simulink model "Vehicle_model"  (R2018a)
settings: Solver=FixedStepAuto  StartTime=0.0  StopTime=40  FixedStep=1e-3  RelTol=1e-2
model workspace (MAT data in the model file):
  Af = 4
  Cd = 0.3
  DrCycles.C505 = [0 1 2 3 4 5 6 7 8 9 10 11 ... (1012 elements, 506x2)]
  DrCycles.FTP = [0 1 2 3 4 5 6 7 8 9 10 11 ... (4956 elements, 2478x2)]
  DrCycles.UDDS = [0 1 2 3 4 5 6 7 8 9 10 11 ... (2746 elements, 1373x2)]
  DrCycles.HWFET = [0 1 2 3 4 5 6 7 8 9 10 11 ... (1532 elements, 766x2)]
  DrCycles.US06 = [0 1 2 3 4 5 6 7 8 9 10 11 ... (1194 elements, 597x2)]
  DrCycles.US06City = [0 1 2 3 4 5 6 7 8 9 10 11 ... (466 elements, 233x2)]
  DrCycles.US06Hwy = [0 1 2 3 4 5 6 7 8 9 10 11 ... (742 elements, 371x2)]
  I = 1
  Kbr = 5000
  P = 20
  Sig = Simulink.Signal
  Sig.DataType = 'auto'
  Sig.Dimensions = -1
  Sig.DimensionsMode = 'auto'
  Sig.Complexity = 'auto'
  Sig.SampleTime = -1
  Sig.SamplingMode = 'auto'
  TimeHWFET = 765
  TimeUDDS = 1372
  TimeUS06 = 596
  axle_b = 10
  axle_k = 5000
  bevAxle_wc = 400
  bevNp = 2
  bevNs = 30
  diffRatio = 3.4
  diffRatio1 = 3.4
  motorMaxTorqueNm = [500 500 500 500 500 500 416.666666667 357.142857143 312.5 277.777777778 250 227.272727273 208.333333333 192.307692308 178.571428571 166.666666667]
  motorMaxTorqueNm2 = [220 220 220 220 220 220 198 176 165 154 143 132 121 110 88 66]
  motorSpeedRadPs = [0 40 80 120 160 200 240 280 320 360 400 440 480 520 560 600]
  motorSpeedRadPs2 = [0 84 168 251 335 419 503 586 670 754 838 922 1005 1089 1173 1361]
  vehicleMass = 1500
  wheelRadius = 0.35
undefined symbols (not defined in the file or in its folder): sigbuilder_block, W_h_o, W_i_h
libraries: simulink x4, autolibdatasheetbattery x2, autolibmappedmotor x2, autolibsharedcoupling x2, autolibshareddiff x2, autolibshared x2, Wheels_Driver_VehDyn_Lib x2
settings Model: PauseTimes=2  Creator=ogden.michael  LastModifiedBy=yassi
settings SolverCC: ZeroCrossAlgorithm=Adaptive
settings DebuggingCC: AlgebraicLoopMsg=none  IgnoredZcDiagnostic=none
settings CodeAppCC: StateflowObjectComments=on
settings SimscapeCC: SimscapeNormalizeSystem=off

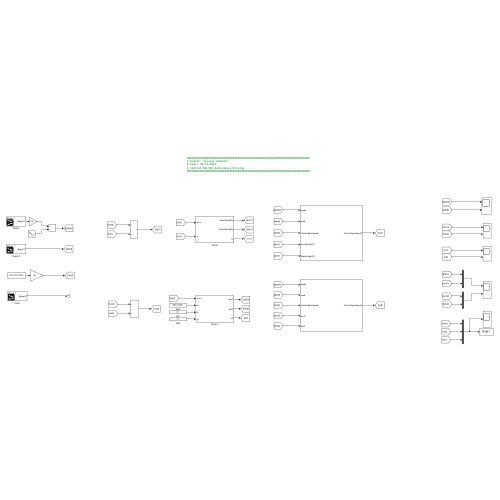
[thumbnail: Simulink's stored preview of the top-level diagram]
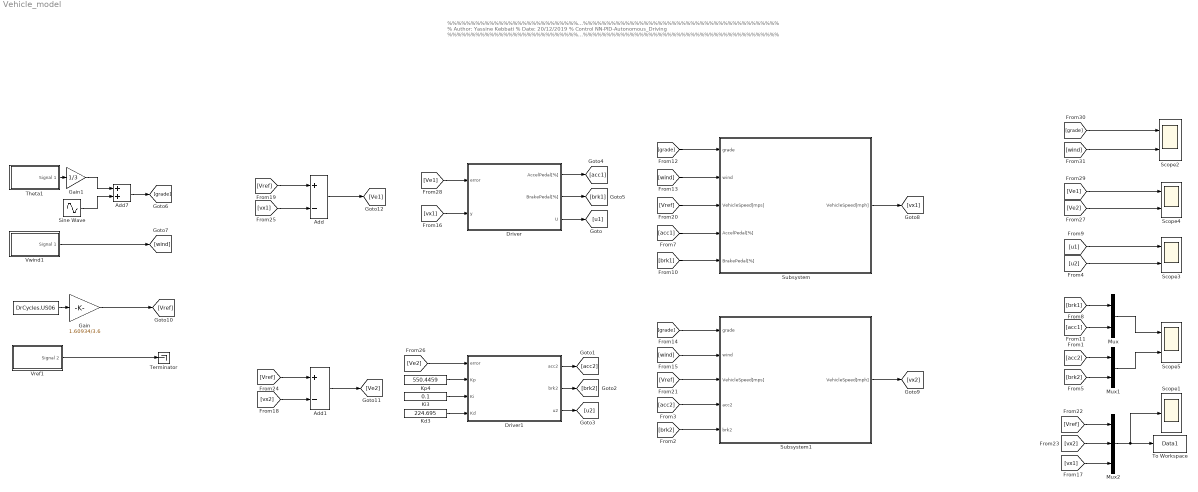
== system Vehicle_model ==
  note: %%%%%%%%%%%%%%%%%%%%%%%%%%%%%%%%%%%%%%%%%%%%%%%%%%%%%%%%%%%%%%%%%%%%%%%%%%%
      | % Author: Yassine Kebbati
      | % Date: 20/12/2019
      | % Control NN-PID-Autonomous_Driving
      | %%%%%%%%%%%%%%%%%%%%%%%%%%%%%%%%%%%%%%%%%%%%%%%%%%%%%%%%%%%%%%%%%%%%%%%%%%%
  " " : FromWorkspace  Tag=DriveCycle  VariableName=DrCycles.US06
  Add : Sum  Inputs=+-
  Add1 : Sum  Inputs=+-
  Add7 : Sum
  Driver : Subsystem  AncestorBlock=Wheels_Driver_VehDyn_Lib/Driver
  Driver1 : Subsystem  AncestorBlock=Wheels_Driver_VehDyn_Lib/Driver
  Gain : Gain  Gain=1.60934/3.6
  Gain1 : Gain  Gain=1/3
  Kd3 : Constant  Value=224.695
  Ki3 : Constant  Value=0.1
  Kp4 : Constant  Value=550.4459
  Mux : Mux  Inputs=2
  Mux1 : Mux  Inputs=2
  Mux2 : Mux  Inputs=3
  Scope1 : Scope
  Scope{2..5} (4 alike) : Scope  NumInputPorts=2
  Sine Wave : Sin  Amplitude=4  Frequency=0.2  SampleTime=0
  Subsystem : Subsystem
  Subsystem1 : Subsystem
  Terminator : Terminator
  Theta1 : Subsystem  Tag=STV Subsys  LoadFcn=sigbuilder_block('load');  StartFcn=sigbuilder_block('start');  StopFcn=sigbuilder_block('stop');  ClipboardFcn=sigbuilder_block('clipboard');  mask(Sigbuilder block){tuvar=[0:10]}
      mask help: Simulink:masks:SigbuilderBlock_MD
      mask init:
      | if ~strcmp(get_param(bdroot(gcbh),'SimulationStatus'),'stopped') tuvar = sigbuilder_block('maskInit'); end
      settings: CopyFcn=sigbuilder_block('copy');  DeleteFcn=sigbuilder_block('delete');  ModelCloseFcn=sigbuilder_block('modelClose');  PreSaveFcn=sigbuilder_block('preSave');  PauseFcn=sigbuilder_block('pause');  ContinueFcn=sigbuilder_block('continue');  NameChangeFcn=sigbuilder_block('namechange');  OpenFcn=sigbuilder_block('open',[6 30 1428 681.75 ]);  CloseFcn=sigbuilder_block('close');
      mask Display: plot(0, 0, 100, 100,[2, 2, 32, 32, 2], [68, 8, 8, 68, 68],[32, 2], [38, 38], [32, 19, 2],[53, 60, 44], [32, 17, 17, 2],[16, 16, 31, 31]);txt = getActiveGroup(gcbh);text(2, 100, txt,'verticalAlignment', 'top');
  To Workspace : ToWorkspace  VariableName=Data1  SaveFormat=Timeseries  SampleTime=-1
  Vref1 : Subsystem  Tag=STV Subsys  LoadFcn=sigbuilder_block('load');  StartFcn=sigbuilder_block('start');  StopFcn=sigbuilder_block('stop');  ClipboardFcn=sigbuilder_block('clipboard');  mask(Sigbuilder block){tuvar=[0:10]}
      mask help: Simulink:masks:SigbuilderBlock_MD
      mask init:
      | if ~strcmp(get_param(bdroot(gcbh),'SimulationStatus'),'stopped') tuvar = sigbuilder_block('maskInit'); end
      settings: CopyFcn=sigbuilder_block('copy');  DeleteFcn=sigbuilder_block('delete');  ModelCloseFcn=sigbuilder_block('modelClose');  PreSaveFcn=sigbuilder_block('preSave');  PauseFcn=sigbuilder_block('pause');  ContinueFcn=sigbuilder_block('continue');  NameChangeFcn=sigbuilder_block('namechange');  OpenFcn=sigbuilder_block('open',[6 51.75 1428 641.25 ]);  CloseFcn=sigbuilder_block('close');
      mask Display: plot(0, 0, 100, 100,[2, 2, 32, 32, 2], [68, 8, 8, 68, 68],[32, 2], [38, 38], [32, 19, 2],[53, 60, 44], [32, 17, 17, 2],[16, 16, 31, 31]);txt = getActiveGroup(gcbh);text(2, 100, txt,'verticalAlignment', 'top');
  Vwind1 : Subsystem  Tag=STV Subsys  LoadFcn=sigbuilder_block('load');  StartFcn=sigbuilder_block('start');  StopFcn=sigbuilder_block('stop');  ClipboardFcn=sigbuilder_block('clipboard');  mask(Sigbuilder block){tuvar=[0:10]}
      mask help: Simulink:masks:SigbuilderBlock_MD
      mask init:
      | if ~strcmp(get_param(bdroot(gcbh),'SimulationStatus'),'stopped') tuvar = sigbuilder_block('maskInit'); end
      settings: CopyFcn=sigbuilder_block('copy');  DeleteFcn=sigbuilder_block('delete');  ModelCloseFcn=sigbuilder_block('modelClose');  PreSaveFcn=sigbuilder_block('preSave');  PauseFcn=sigbuilder_block('pause');  ContinueFcn=sigbuilder_block('continue');  NameChangeFcn=sigbuilder_block('namechange');  OpenFcn=sigbuilder_block('open',[6 30 1428 681.75 ]);  CloseFcn=sigbuilder_block('close');
      mask Display: plot(0, 0, 100, 100,[2, 2, 32, 32, 2], [68, 8, 8, 68, 68],[32, 2], [38, 38], [32, 19, 2],[53, 60, 44], [32, 17, 17, 2],[16, 16, 31, 31]);txt = getActiveGroup(gcbh);text(2, 100, txt,'verticalAlignment', 'top');
  wires:
  [grade] -> Subsystem/1(grade)
  Sine Wave/1 -> Add7/2
  Theta1/1(Signal 1) -> Gain1/1
  [Ve1] -> Driver/1(" error")
  Gain1/1 -> Add7/1
  [wind] -> Subsystem/2(wind)
  Kp4/1 -> Driver1/2(Kp)
  Ki3/1 -> Driver1/3(Ki)
  Kd3/1 -> Driver1/4(Kd)
  Mux/1 -> Scope5/1
  Mux1/1 -> Scope5/2
  [Ve2] -> Scope4/2
  Mux2/1 -> To Workspace/1, Scope1/1
  [vx2] -> Add1/2
  [vx1] -> Driver/2(" y")
  [Vref] -> Add/1
  Vwind1/1(Signal 1) -> [wind]
  Add7/1 -> [grade]
  Driver1/1(acc2) -> [acc2]
  Driver1/2(brk2) -> [brk2]
  [acc2] -> Subsystem1/4(acc2)
  [acc2] -> Mux1/1
  [brk2] -> Subsystem1/5(brk2)
  [brk2] -> Mux1/2
  [u2] -> Scope3/2
  Driver1/3(u2) -> [u2]
  Driver/3(U) -> [u1]
  [u1] -> Scope3/1
  Driver/2(BrakePedal[%]) -> [brk1]
  [brk1] -> Mux/1
  [brk1] -> Subsystem/5(BrakePedal[%])
  Driver/1(AccelPedal[%]) -> [acc1]
  [acc1] -> Subsystem/4(AccelPedal[%])
  [acc1] -> Mux/2
  [grade] -> Subsystem1/1(grade)
  [wind] -> Subsystem1/2(wind)
  Subsystem/1(VehicleSpeed[mph]) -> [vx1]
  [vx1] -> Mux2/3
  Subsystem1/1(VehicleSpeed[mph]) -> [vx2]
  [Vref] -> Subsystem/3(VehicleSpeed[mps])
  [Vref] -> Subsystem1/3(VehicleSpeed[mps])
  [Vref] -> Mux2/1
  [vx2] -> Mux2/2
  [Vref] -> Add1/1
  [vx1] -> Add/2
  Add1/1 -> [Ve2]
  [Ve2] -> Driver1/1(" error")
  Add/1 -> [Ve1]
  [Ve1] -> Scope4/1
  [grade] -> Scope2/1
  [wind] -> Scope2/2
  " "/1 -> Gain/1
  Vref1/1(Signal 2) -> Terminator/1
  Gain/1 -> [Vref]

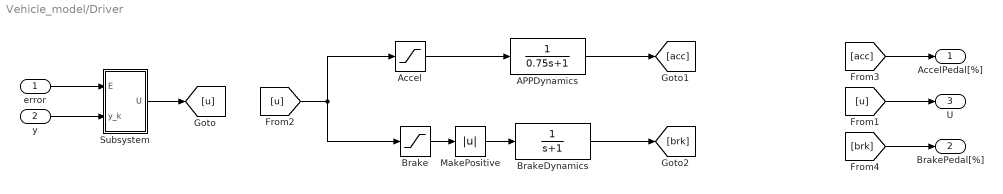
== system Vehicle_model/Driver ==
  " error" : Inport
  " y" : Inport  Port=2
  APPDynamics : TransferFcn  Denominator=[0.75 1]
  Accel : Saturate  UpperLimit=100  LowerLimit=0
  Brake : Saturate  UpperLimit=0  LowerLimit=-100
  BrakeDynamics : TransferFcn  Denominator=[1 1]
  MakePositive : Abs
  Subsystem : Subsystem
  AccelPedal[%] : Outport  VectorParamsAs1DForOutWhenUnconnected=off
  BrakePedal[%] : Outport  Port=2  VectorParamsAs1DForOutWhenUnconnected=off
  U : Outport  Port=3  VectorParamsAs1DForOutWhenUnconnected=off
  wires:
  MakePositive/1 -> BrakeDynamics/1
  " error"/1 -> Subsystem/1(E)
  Accel/1 -> APPDynamics/1
  Brake/1 -> MakePositive/1
  " y"/1 -> Subsystem/2(y_k)
  BrakeDynamics/1 -> [brk]
  APPDynamics/1 -> [acc]
  [u] -> Accel/1, Brake/1
  Subsystem/1(U) -> [u]
  [u] -> U/1
  [acc] -> AccelPedal[%]/1
  [brk] -> BrakePedal[%]/1

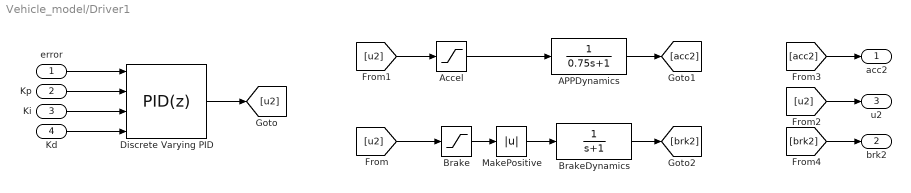
== system Vehicle_model/Driver1 ==
  " error" : Inport
  Kp : Inport  Port=2
  Ki : Inport  Port=3
  Kd : Inport  Port=4
  APPDynamics : TransferFcn  Denominator=[0.75 1]
  Accel : Saturate  UpperLimit=100  LowerLimit=0
  Brake : Saturate  UpperLimit=0  LowerLimit=-100
  BrakeDynamics : TransferFcn  Denominator=[1 1]
  Discrete Varying PID : simulink/Continuous/PID Controller  Controller=PID  Form=Parallel  TimeDomain=Discrete-time  SampleTime=-1  IntegratorMethod=Forward Euler  ControllerParametersSource=external  P=1  I=1  D=0  N=100  UseFilter=off  TunerSelectOption=Transfer Function Based (PID Tuner App)  InitialConditionSource=internal  InitialConditionForIntegrator=0  InitialConditionForFilter=0  DifferentiatorICPrevScaledInput=0  ExternalReset=none  TrackingMode=off  Kt=1  LimitOutput=off  UpperSaturationLimit=100  LowerSaturationLimit=-100  LinearizeAsGain=on  AntiWindupMode=none  Kb=1  POutMin=[]  POutMax=[]  IOutMin=[]  IOutMax=[]  DOutMin=[]  DOutMax=[]  NOutMin=[]  NOutMax=[]  SumOutMin=[]  SumOutMax=[]  SaturationOutMin=[]  SaturationOutMax=[]  PParamMin=[]  PParamMax=[]  IParamMin=[]  IParamMax=[]  DParamMin=[]  DParamMax=[]  NParamMin=[]  NParamMax=[]  KbParamMin=[]  KbParamMax=[]  KtParamMin=[]  KtParamMax=[]  KbOutMin=[]  KbOutMax=[]  KtOutMin=[]  KtOutMax=[]  IntegratorOutMin=[]  IntegratorOutMax=[]  FilterOutMin=[]  FilterOutMax=[]  SumI1OutMin=[]  SumI1OutMax=[]  SumI2OutMin=[]  SumI2OutMax=[]  SumI3OutMin=[]  SumI3OutMax=[]  SumDOutMin=[]  SumDOutMax=[]  DifferentiatorOutMin=[]  DifferentiatorOutMax=[]  FilterDiffOutCoefMin=[]  FilterDiffOutCoefMax=[]  ReciprocalOutMin=[]  ReciprocalOutMax=[]  SumDenOutMin=[]  SumDenOutMax=[]  SumNumOutMin=[]  SumNumOutMax=[]  DivideOutMin=[]  DivideOutMax=[]  IntegratorContinuousStateAttributes=''  IntegratorStateMustResolveToSignalObject=off  IntegratorRTWStateStorageClass=Auto  FilterContinuousStateAttributes=''  FilterStateMustResolveToSignalObject=off  FilterRTWStateStorageClass=Auto
  MakePositive : Abs
  acc2 : Outport  VectorParamsAs1DForOutWhenUnconnected=off
  brk2 : Outport  Port=2  VectorParamsAs1DForOutWhenUnconnected=off
  u2 : Outport  Port=3  VectorParamsAs1DForOutWhenUnconnected=off
  wires:
  MakePositive/1 -> BrakeDynamics/1
  " error"/1 -> Discrete Varying PID/1
  Accel/1 -> APPDynamics/1
  Kp/1 -> Discrete Varying PID/2
  Kd/1 -> Discrete Varying PID/4
  Ki/1 -> Discrete Varying PID/3
  Brake/1 -> MakePositive/1
  BrakeDynamics/1 -> [brk2]
  APPDynamics/1 -> [acc2]
  Discrete Varying PID/1 -> [u2]
  [u2] -> Brake/1
  [u2] -> Accel/1
  [u2] -> u2/1
  [acc2] -> acc2/1
  [brk2] -> brk2/1

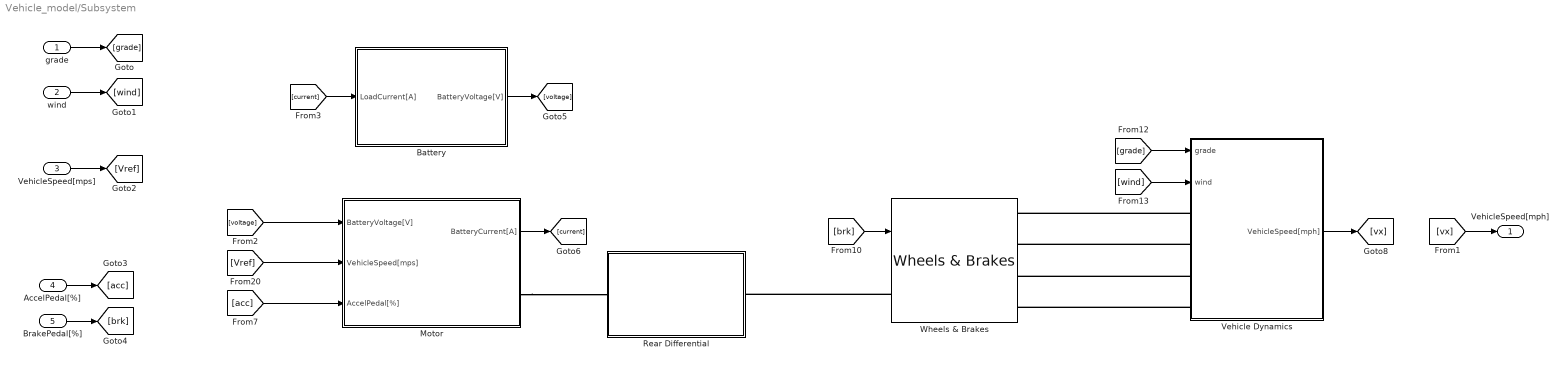
== system Vehicle_model/Subsystem ==
  grade : Inport
  wind : Inport  Port=2
  VehicleSpeed[mps] : Inport  Port=3
  AccelPedal[%] : Inport  Port=4
  BrakePedal[%] : Inport  Port=5
  Battery : Subsystem
  Motor : Subsystem
  Rear Differential : Subsystem
  Vehicle Dynamics : Subsystem  AncestorBlock=Wheels_Driver_VehDyn_Lib/Vehicle Dynamics
  "Wheels & Brakes " : Wheels_Driver_VehDyn_Lib/Wheels & Brakes  SystemSampleTime=-1  Latency=0  AutoFrameSizeCalculation=off
      link override BrakeGain: Gain=Kbr
      link override Longitudinal Wheel - Disk Brake: Re=0.32995  Lrel=0.32995  rollingType=Magic Formula  Iyy=0.798  UNLOADED_RADIUS=0.32995  num_pads=2
      link override Longitudinal Wheel - Disk Brake1: Iyy=0.798  Lrel=0.32995  Re=0.32995  rollingType=Magic Formula  UNLOADED_RADIUS=0.32995
  VehicleSpeed[mph] : Outport
  wires:
  [wind] -> Vehicle Dynamics/2(wind)
  [current] -> Battery/1(LoadCurrent[A])
  [voltage] -> Motor/1(BatteryVoltage[V])
  [grade] -> Vehicle Dynamics/1(grade)
  [vx] -> VehicleSpeed[mph]/1
  [brk] -> "Wheels & Brakes "/1
  [Vref] -> Motor/2(VehicleSpeed[mps])
  [acc] -> Motor/3(AccelPedal[%])
  Vehicle Dynamics/1(VehicleSpeed[mph]) -> [vx]
  grade/1 -> [grade]
  wind/1 -> [wind]
  VehicleSpeed[mps]/1 -> [Vref]
  AccelPedal[%]/1 -> [acc]
  BrakePedal[%]/1 -> [brk]
  Battery/1(BatteryVoltage[V]) -> [voltage]
  Motor/1(BatteryCurrent[A]) -> [current]
  connections:
  Motor/RConn1 -- Rear Differential/LConn1
  Vehicle Dynamics/LConn4 -- "Wheels & Brakes "/RConn4
  Vehicle Dynamics/LConn2 -- "Wheels & Brakes "/RConn2
  Vehicle Dynamics/LConn1 -- "Wheels & Brakes "/RConn1
  Vehicle Dynamics/LConn3 -- "Wheels & Brakes "/RConn3
  "Wheels & Brakes "/LConn1 -- Rear Differential/RConn1

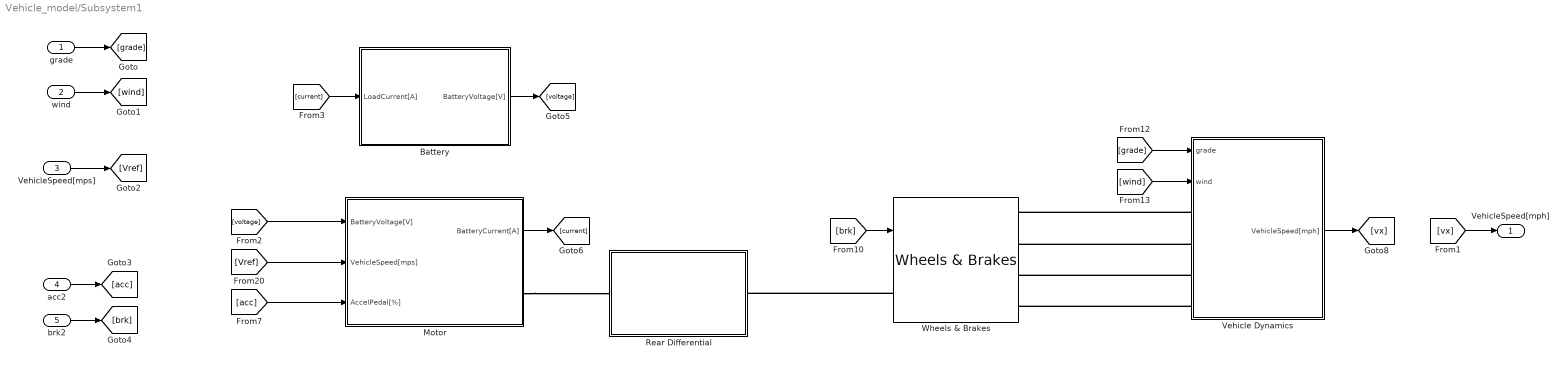
== system Vehicle_model/Subsystem1 ==
  grade : Inport
  wind : Inport  Port=2
  VehicleSpeed[mps] : Inport  Port=3
  acc2 : Inport  Port=4
  brk2 : Inport  Port=5
  Battery : Subsystem
  Motor : Subsystem
  Rear Differential : Subsystem
  Vehicle Dynamics : Subsystem  AncestorBlock=Wheels_Driver_VehDyn_Lib/Vehicle Dynamics
  "Wheels & Brakes " : Wheels_Driver_VehDyn_Lib/Wheels & Brakes  SystemSampleTime=-1  Latency=0  AutoFrameSizeCalculation=off
      link override BrakeGain: Gain=Kbr
      link override Longitudinal Wheel - Disk Brake: Re=0.32995  Lrel=0.32995  rollingType=Magic Formula  Iyy=0.798  UNLOADED_RADIUS=0.32995  num_pads=2
      link override Longitudinal Wheel - Disk Brake1: Iyy=0.798  Lrel=0.32995  Re=0.32995  rollingType=Magic Formula  UNLOADED_RADIUS=0.32995
  VehicleSpeed[mph] : Outport
  wires:
  [vx] -> VehicleSpeed[mph]/1
  wind/1 -> [wind]
  [Vref] -> Motor/2(VehicleSpeed[mps])
  [grade] -> Vehicle Dynamics/1(grade)
  [acc] -> Motor/3(AccelPedal[%])
  [current] -> Battery/1(LoadCurrent[A])
  VehicleSpeed[mps]/1 -> [Vref]
  brk2/1 -> [brk]
  Motor/1(BatteryCurrent[A]) -> [current]
  [voltage] -> Motor/1(BatteryVoltage[V])
  Vehicle Dynamics/1(VehicleSpeed[mph]) -> [vx]
  [brk] -> "Wheels & Brakes "/1
  [wind] -> Vehicle Dynamics/2(wind)
  grade/1 -> [grade]
  acc2/1 -> [acc]
  Battery/1(BatteryVoltage[V]) -> [voltage]
  connections:
  Motor/RConn1 -- Rear Differential/LConn1
  Vehicle Dynamics/LConn4 -- "Wheels & Brakes "/RConn4
  Vehicle Dynamics/LConn3 -- "Wheels & Brakes "/RConn3
  "Wheels & Brakes "/LConn1 -- Rear Differential/RConn1
  Vehicle Dynamics/LConn1 -- "Wheels & Brakes "/RConn1
  Vehicle Dynamics/LConn2 -- "Wheels & Brakes "/RConn2

== system Vehicle_model/Theta1 ==
  Demux : Demux  Tag=STV Demux  Outputs=1
      settings: DisplayOption=none
  FromWs : FromWorkspace  Tag=STV FromWs  VariableName=tuvar
      SigBuilderData=|
      | common.afterFinalStr = 'Extrapolate'
      | common.sampleTime = 0
      | dataSet.timeRange = [0 100]
      | dataSet.name = 'Group 1'
      | sbobj.Groups.Name = 'Group 1'
      | sbobj.Groups.Signals.Name = 'Signal 1'
      | sbobj.Groups.Signals.XData = [0 1 2 3 4 5 6 7 8 9 10 11 12 13 14 15 16 17 18 19 20 21 22 23 24 25 26 27 28 29 30 31 32 33 34 35 36 37 38 39 40 41 42 43 44 45 46 47 48 49 50 51 52 53 54 55 56 57 58 59 60 61 62 63 64 65 66 67 68 69 70 71 72 73 74 75 76 77 78 79 80 81 82 83 84 85 86 87 88 89 90 91 92 93 94 95 96 97 98 100]
      | sbobj.Groups.Signals.YData = [0 0 0 0 0 0 0 0.05 0.15 0.2 0.5 1 2 3 4 5 6 7 8 9 10 11 12 13 14 14.5 14.8 15 15 15 15 15 15 15 14.95 14.7 14.45 14.1 13.15 11.85 11 9.95 8.7 8.15 7.35 6 4.6 3.55 2.25 1.35 0.75 0.15 0 0 0 0 0 0 0 0 -0.15 -0.4 -1.15 -2 -3 -4 -5 -6 -6.65 -7.45 -7.9 -8 -8 -8 -8 -8 -8 -8 -8 -8 -7.8 -7.55 -7.45 -7.15 -6.85 -6.5 -6 -5.5 -5.25 -5.2 -5.2 -5.15 -5 -5 -5 -5 -5 -5 -5 -5]
      | sbobj.Groups.TimeRange = [0 100]
  Signal 1 : Outport  Tag=STV Outport
  wires:
  Demux/1 -> Signal 1/1
  FromWs/1 -> Demux/1

== system Vehicle_model/Vref1 ==
  Demux : Demux  Tag=STV Demux  Outputs=1
      settings: DisplayOption=none
  FromWs : FromWorkspace  Tag=STV FromWs  VariableName=tuvar
      SigBuilderData=|
      | common.afterFinalStr = 'Extrapolate'
      | common.sampleTime = 0
      | dataSet.timeRange = [0 99]
      | dataSet.name = 'Group 1'
      | sbobj.Groups.Name = 'Group 1'
      | sbobj.Groups.Signals.Name = 'Signal 2'
      | sbobj.Groups.Signals.XData = [0 1 2 3 4 5 6 7 8 9 10 11 12 13 14 15 16 17 18 19 20 21 22 23 24 25 26 27 28 29 30 31 32 33 34 35 36 37 38 39 40 41 42 43 44 45 46 47 48 49 50 51 52 53 54 55 56 57 58 59 60 61 62 63 64 65 66 67 68 69 70 71 72 73 74 75 76 77 78 79 80 81 82 83 84 85 86 87 88 89 90 91 92 93 94 95 96 97 98 99]
      | sbobj.Groups.Signals.YData = [5 5 5 5 5 5 5 5 5 5 5 5 5 5 5 5 5 5 5 5 15 15 15 15 15 15 15 15 15 15 15 15 15 15 15 15 15 15 15 15 30 30 30 30 30 30 30 30 30 30 30 30 30 30 30 30 30 30 30 30 20 20 20 20 20 20 20 20 20 20 20 20 20 20 20 20 20 20 20 20 10 10 10 10 10 10 10 10 10 10 10 10 10 10 10 10 10 10 10 10]
      | sbobj.Groups.TimeRange = [0 99]
  Signal 2 : Outport  Tag=STV Outport
  wires:
  FromWs/1 -> Demux/1
  Demux/1 -> Signal 2/1

== system Vehicle_model/Vwind1 ==
  Demux : Demux  Tag=STV Demux  Outputs=1
      settings: DisplayOption=none
  FromWs : FromWorkspace  Tag=STV FromWs  VariableName=tuvar
      SigBuilderData=|
      | common.afterFinalStr = 'Extrapolate'
      | common.sampleTime = 0
      | dataSet.timeRange = [0 100]
      | dataSet.name = 'Group 1'
      | sbobj.Groups.Name = 'Group 1'
      | sbobj.Groups.Signals.Name = 'Signal 1'
      | sbobj.Groups.Signals.XData = [0 1 2 3 4 5 6 7 8 9 10 11 12 13 14 15 16 17 18 19 20 21 22 23 24 25 26 27 28 29 30 31 32 33 34 35 36 37 38 39 40 41 42 43 44 45 46 47 48 49 50 51 52 53 54 55 56 57 58 59 60 61 62 63 64 65 66 67 68 69 70 71 72 73 74 75 76 77 78 79 80 81 82 83 84 85 86 87 88 89 90 91 92 93 94 95 96 97 98 100]
      | sbobj.Groups.Signals.YData = [-8 -8 -8 -8 -8 -8 -8 -8 -8 -8 -8 -8 -8 -8 -8 -8 -8 -8 -8 -8 -2 -2 -2 -2 -2 -2 -2 -2 -2 -2 -2 -2 -2 -2 -2 -2 -2 -2 -2 -2 10 10 10 10 10 10 10 10 10 10 10 10 10 10 10 10 10 10 10 10 15 15 15 15 15 15 15 15 15 15 15 15 15 15 15 15 15 15 15 15 5 5 5 5 5 5 5 5 5 5 5 5 5 5 5 5 5 5 5 5]
      | sbobj.Groups.TimeRange = [0 100]
  Signal 1 : Outport  Tag=STV Outport
  wires:
  FromWs/1 -> Demux/1
  Demux/1 -> Signal 1/1

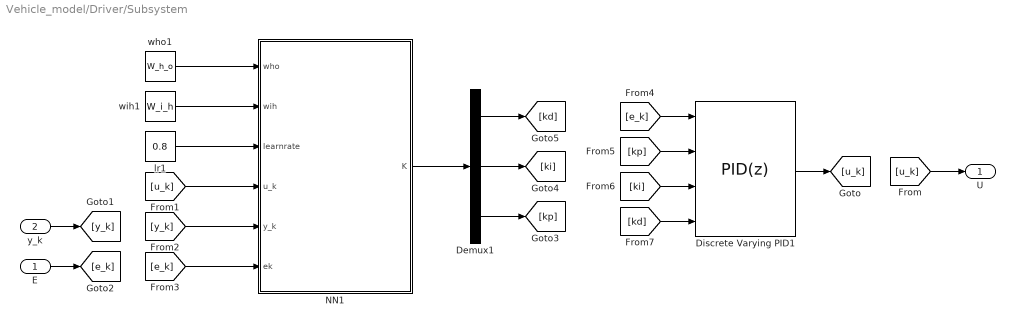
== system Vehicle_model/Driver/Subsystem ==
  E : Inport
  y_k : Inport  Port=2
  Demux1 : Demux  Outputs=3
  Discrete Varying PID1 : simulink/Continuous/PID Controller  Controller=PID  Form=Parallel  TimeDomain=Discrete-time  SampleTime=-1  IntegratorMethod=Forward Euler  ControllerParametersSource=external  P=1  I=1  D=0  N=100  UseFilter=off  TunerSelectOption=Transfer Function Based (PID Tuner App)  InitialConditionSource=internal  InitialConditionForIntegrator=0  InitialConditionForFilter=0  DifferentiatorICPrevScaledInput=0  ExternalReset=none  TrackingMode=off  Kt=1  LimitOutput=off  UpperSaturationLimit=100  LowerSaturationLimit=-100  LinearizeAsGain=on  AntiWindupMode=none  Kb=1  POutMin=[]  POutMax=[]  IOutMin=[]  IOutMax=[]  DOutMin=[]  DOutMax=[]  NOutMin=[]  NOutMax=[]  SumOutMin=[]  SumOutMax=[]  SaturationOutMin=[]  SaturationOutMax=[]  PParamMin=[]  PParamMax=[]  IParamMin=[]  IParamMax=[]  DParamMin=[]  DParamMax=[]  NParamMin=[]  NParamMax=[]  KbParamMin=[]  KbParamMax=[]  KtParamMin=[]  KtParamMax=[]  KbOutMin=[]  KbOutMax=[]  KtOutMin=[]  KtOutMax=[]  IntegratorOutMin=[]  IntegratorOutMax=[]  FilterOutMin=[]  FilterOutMax=[]  SumI1OutMin=[]  SumI1OutMax=[]  SumI2OutMin=[]  SumI2OutMax=[]  SumI3OutMin=[]  SumI3OutMax=[]  SumDOutMin=[]  SumDOutMax=[]  DifferentiatorOutMin=[]  DifferentiatorOutMax=[]  FilterDiffOutCoefMin=[]  FilterDiffOutCoefMax=[]  ReciprocalOutMin=[]  ReciprocalOutMax=[]  SumDenOutMin=[]  SumDenOutMax=[]  SumNumOutMin=[]  SumNumOutMax=[]  DivideOutMin=[]  DivideOutMax=[]  IntegratorContinuousStateAttributes=''  IntegratorStateMustResolveToSignalObject=off  IntegratorRTWStateStorageClass=Auto  FilterContinuousStateAttributes=''  FilterStateMustResolveToSignalObject=off  FilterRTWStateStorageClass=Auto
  NN1 : Subsystem
  lr1 : Constant  Value=0.8  SampleTime=-1
  who1 : Constant  Value=W_h_o  SampleTime=-1
  wih1 : Constant  Value=W_i_h  SampleTime=-1
  U : Outport
  wires:
  lr1/1 -> NN1/3(learnrate)
  who1/1 -> NN1/1(who)
  [u_k] -> U/1
  wih1/1 -> NN1/2(wih)
  [e_k] -> NN1/6(ek)
  NN1/1(K) -> Demux1/1
  [y_k] -> NN1/5(y_k)
  Discrete Varying PID1/1 -> [u_k]
  [u_k] -> NN1/4(u_k)
  E/1 -> [e_k]
  y_k/1 -> [y_k]
  [e_k] -> Discrete Varying PID1/1
  Demux1/3 -> [kp]
  Demux1/2 -> [ki]
  Demux1/1 -> [kd]
  [kp] -> Discrete Varying PID1/2
  [ki] -> Discrete Varying PID1/3
  [kd] -> Discrete Varying PID1/4

== system Vehicle_model/Subsystem/Battery ==
  LoadCurrent[A] : Inport
  AmbientTemp[C] : Constant  Value=27
  Bus Selector : BusSelector  OutputSignals=BattSoc
  C2K : Bias  Bias=273
  Datasheet Battery : autolibdatasheetbattery/Datasheet Battery  CapacityCtrl=Parameter  OutputVlt=Unfiltered  BattChargeMax=131.82  Em=[3.167 3.413 3.446 3.488 3.537 3.571 3.593 3.610 3.625 3.642 3.663 3.695 3.755 3.799 3.846 3.895 3.945 3.997 4.051 4.108 4.166]  CapLUTBp=[0 0.05 0.1 0.15 0.2 0.25 0.3 0.35 0.4 0.45 0.5 0.55 0.6 0.65 0.7 0.75 0.8 0.85 0.9 0.95 1]  RInt=[0.008846 0.009319 0.009027 0.00847 0.01032 0.01314;0.006389 0.006554 0.005553 0.005525 0.006043 0.007805;0.004364 0.004101 0.00406 0.003452 0.003846 0.004517;0.002031 0.002563 0.002532 0.00246 0.002716 0.003047;0.001443 0.001825 0.001795 0.001778 0.001924 0.002234;0.0005603 0.0007192 0.0006887 0.0007557 0.0007355 0.001014;0.001028 0.001338 0.001 0.001536 0.001546 0.002789]  BattTempBp=[243.1 253.1 263.1 273.1 283.1 298.1 313.1]  CapSOCBp=[0 0.2 0.4 0.6 0.8 1]  Ns=96  Np=2  BattCapInit=131.82  Tc=1/1000  Vinit=4.221
  SOCto% : Gain  Gain=100
  Scope : Scope
  Stop Simulation : Stop
  lowSOClimit : simulink/Logic and Bit Operations/Compare To Constant  relop=<=  const=5  OutDataTypeStr=boolean
  BatteryVoltage[V] : Outport  VectorParamsAs1DForOutWhenUnconnected=off
  wires:
  Datasheet Battery/1 -> Bus Selector/1
  AmbientTemp[C]/1 -> C2K/1
  Datasheet Battery/2 -> BatteryVoltage[V]/1
  C2K/1 -> Datasheet Battery/2
  SOCto%/1 -> lowSOClimit/1, Scope/1
  Bus Selector/1 -> SOCto%/1  "<BattSoc>"
  LoadCurrent[A]/1 -> Datasheet Battery/1
  lowSOClimit/1 -> Stop Simulation/1

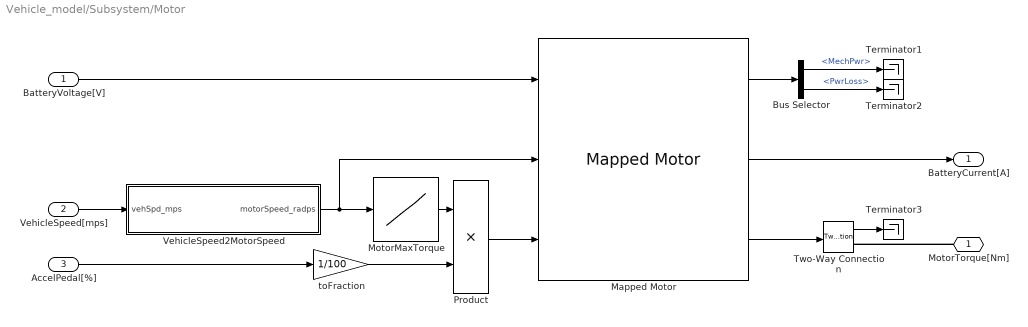
== system Vehicle_model/Subsystem/Motor ==
  BatteryVoltage[V] : Inport
  VehicleSpeed[mps] : Inport  Port=2
  AccelPedal[%] : Inport  Port=3
  Bus Selector : BusSelector  OutputSignals=MechPwr,PwrLoss
  Mapped Motor : autolibmappedmotor/Mapped Motor  port_config=Speed  param_by=Tabulated torque-speed envelope  w_t=motorSpeedRadPs  T_t=motorMaxTorqueNm  torque_max=.1  power_max=30  Tc=0.02  param_loss=Single efficiency measurement  eff=100  w_eff=375  T_eff=0.08  Piron=0  Pbase=0  w_eff_bp=[-8000 -4000 0 4000 8000]  T_eff_bp=[0 0.03 0.06 0.09]  losses_table=[1.49 1.67 2.21 3.10; 0.42 0.69 1.14 2.03; 0.06 0.24 0.78 1.68; 0.42 0.69 1.14 2.03; 1.49 1.67 2.21 3.10]  efficiency_table=[95 95 95 95; 95 95 95 95; 95 95 95 95; 95 95 95 95; 95 95 95 95]  J=5e-6  b=1e-5  omega_o=0  T_t_extended=[166.666666666667 178.571428571429 192.307692307692 208.333333333333 227.272727272727 250 277.777777777778 312.5 357.142857142857 416.666666666667 500 500 500 500 500 500 500 500 500 500 500 416.666666666667 357.142857142857 312.5 277.777777777778 250 227.272727272727 208.333333333333 192.307692307692 178.571428571429 166.666666666667]  w_t_extended=[-600 -560 -520 -480 -440 -400 -360 -320 -280 -240 -200 -160 -120 -80 -40 0 40 80 120 160 200 240 280 320 360 400 440 480 520 560 600]  KLossIron=0  KLossCopper=0  x_w_eff_vec=[-8000 -4000 0 4000 8000]  x_T_eff_vec=[-0.09 -0.06 -0.03 0 0.03 0.06 0.09]  x_losses_mat=[3.1 2.21 1.67 1.49 1.67 2.21 3.1;2.03 1.14 0.69 0.42 0.69 1.14 2.03;1.68 0.78 0.24 0.06 0.24 0.78 1.68;2.03 1.14 0.69 0.42 0.69 1.14 2.03;3.1 2.21 1.67 1.49 1.67 2.21 3.1]  aMode=aMode
  MotorMaxTorque : Lookup_n-D  NumberOfTableDimensions=1  BreakpointsForDimension1=motorSpeedRadPs  Table=motorMaxTorqueNm  ExtrapMethod=Clip  InternalRulePriority=Speed  RndMeth=Simplest  InputSameDT=on
  Product : Product
  Terminator1 : Terminator
  Terminator2 : Terminator
  Terminator3 : Terminator
  Two-Way Connectio n : TwoWayConnection
  VehicleSpeed2MotorSpeed : Subsystem
  toFraction : Gain  Gain=1/100
  MotorTorque[Nm] : PMIOPort  Side=Right
  BatteryCurrent[A] : Outport  VectorParamsAs1DForOutWhenUnconnected=off
  wires:
  BatteryVoltage[V]/1 -> Mapped Motor/1
  Mapped Motor/2 -> BatteryCurrent[A]/1
  VehicleSpeed[mps]/1 -> VehicleSpeed2MotorSpeed/1(vehSpd_mps)
  VehicleSpeed2MotorSpeed/1(motorSpeed_radps) -> MotorMaxTorque/1, Mapped Motor/2
  Mapped Motor/1 -> Bus Selector/1
  Two-Way Connectio n/1 -> Terminator3/1
  Product/1 -> Mapped Motor/3
  MotorMaxTorque/1 -> Product/1
  AccelPedal[%]/1 -> toFraction/1
  toFraction/1 -> Product/2
  Bus Selector/2 -> Terminator2/1  "<PwrLoss>"
  Bus Selector/1 -> Terminator1/1  "<MechPwr>"
  Mapped Motor/3 -> Two-Way Connectio n/1
  connections:
  MotorTorque[Nm]/RConn1 -- Two-Way Connectio n/RConn1

== system Vehicle_model/Subsystem/Rear Differential ==
  Axle : autolibsharedcoupling/Torsional Compliance  port_config=Two-way connection  k=axle_k  b=axle_b  theta_o=0  domega_o=0  omega_c=bevAxle_wc  blkID=0  aMode=1
  Open Differential : autolibshareddiff/Open Differential  shaftSwitchMask=To the left of center-line  Ndiff=diffRatio  Jd=.025  bd=1e-3  Jw1=.01  bw1=1e-3  Jw2=.01  bw2=1e-3  omegaw1o=0  omegaw2o=0  maxAbsSpd=5e3  aMode=aMode
  Terminator5 : Terminator
  Terminator6 : Terminator
  Two-Way Connection1 : TwoWayConnection
  Two-Way Connection2 : TwoWayConnection
  AxleTorque[Nm] : PMIOPort  Side=Right
  TorqueInput[Nm] : PMIOPort  Port=2  Side=Left
  wires:
  Open Differential/3 -> Two-Way Connection1/1
  Open Differential/4 -> Terminator5/1
  Open Differential/1 -> Terminator6/1  "Diff"
  Open Differential/2 -> Two-Way Connection2/1
  Two-Way Connection1/1 -> Open Differential/2, Open Differential/3
  Two-Way Connection2/1 -> Open Differential/1
  connections:
  Axle/LConn1 -- Two-Way Connection1/RConn1
  TorqueInput[Nm]/RConn1 -- Two-Way Connection2/RConn1
  AxleTorque[Nm]/RConn1 -- Axle/RConn1

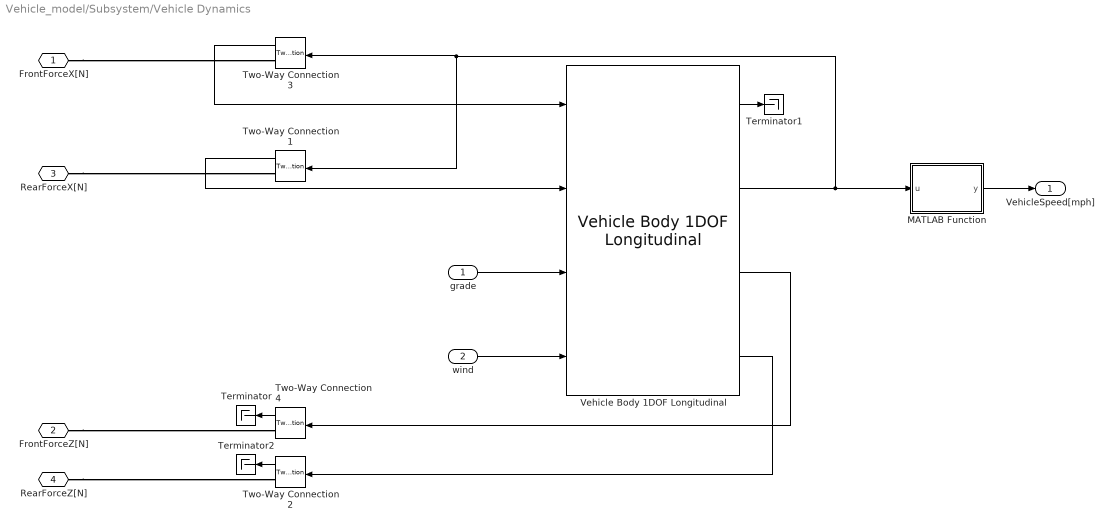
== system Vehicle_model/Subsystem/Vehicle Dynamics ==
  grade : Inport
  wind : Inport  Port=2
  MATLAB Function : MATLAB Function  TreatAsAtomicUnit=on
  Terminator : Terminator
  Terminator1 : Terminator
  Terminator2 : Terminator
  Two-Way Connection{1..4} (4 alike) : TwoWayConnection
  Vehicle Body 1DOF Longitudinal : autolibshared/Vehicle Body 1DOF Longitudinal  VariantControl=SL  aMode=aMode  NF=2  NR=2  m=1468  a=1.13225  b=1.45575  h=.35  Cd=0.29  Af=2.22  x_o=0  xdot_o=0  Pabs=101325  T=293.15  g=9.81
  FrontForceX[N] : PMIOPort  Side=Left
  FrontForceZ[N] : PMIOPort  Port=2  Side=Left
  RearForceX[N] : PMIOPort  Port=3  Side=Left
  RearForceZ[N] : PMIOPort  Port=4  Side=Left
  VehicleSpeed[mph] : Outport  VectorParamsAs1DForOutWhenUnconnected=off
  wires:
  grade/1 -> Vehicle Body 1DOF Longitudinal/3
  wind/1 -> Vehicle Body 1DOF Longitudinal/4
  Vehicle Body 1DOF Longitudinal/1 -> Terminator1/1
  Vehicle Body 1DOF Longitudinal/3 -> Two-Way Connection4/1
  Vehicle Body 1DOF Longitudinal/4 -> Two-Way Connection2/1
  Two-Way Connection3/1 -> Vehicle Body 1DOF Longitudinal/1
  Two-Way Connection1/1 -> Vehicle Body 1DOF Longitudinal/2
  Two-Way Connection4/1 -> Terminator/1
  Two-Way Connection2/1 -> Terminator2/1
  Vehicle Body 1DOF Longitudinal/2 -> MATLAB Function/1(u), Two-Way Connection1/1, Two-Way Connection3/1
  MATLAB Function/1(y) -> VehicleSpeed[mph]/1
  connections:
  FrontForceX[N]/RConn1 -- Two-Way Connection3/RConn1
  FrontForceZ[N]/RConn1 -- Two-Way Connection4/RConn1
  RearForceX[N]/RConn1 -- Two-Way Connection1/RConn1
  RearForceZ[N]/RConn1 -- Two-Way Connection2/RConn1

== system Vehicle_model/Subsystem1/Battery ==
  LoadCurrent[A] : Inport
  AmbientTemp[C] : Constant  Value=27
  Bus Selector : BusSelector  OutputSignals=BattSoc
  C2K : Bias  Bias=273
  Datasheet Battery : autolibdatasheetbattery/Datasheet Battery  CapacityCtrl=Parameter  OutputVlt=Unfiltered  BattChargeMax=131.82  Em=[3.167 3.413 3.446 3.488 3.537 3.571 3.593 3.610 3.625 3.642 3.663 3.695 3.755 3.799 3.846 3.895 3.945 3.997 4.051 4.108 4.166]  CapLUTBp=[0 0.05 0.1 0.15 0.2 0.25 0.3 0.35 0.4 0.45 0.5 0.55 0.6 0.65 0.7 0.75 0.8 0.85 0.9 0.95 1]  RInt=[0.008846 0.009319 0.009027 0.00847 0.01032 0.01314;0.006389 0.006554 0.005553 0.005525 0.006043 0.007805;0.004364 0.004101 0.00406 0.003452 0.003846 0.004517;0.002031 0.002563 0.002532 0.00246 0.002716 0.003047;0.001443 0.001825 0.001795 0.001778 0.001924 0.002234;0.0005603 0.0007192 0.0006887 0.0007557 0.0007355 0.001014;0.001028 0.001338 0.001 0.001536 0.001546 0.002789]  BattTempBp=[243.1 253.1 263.1 273.1 283.1 298.1 313.1]  CapSOCBp=[0 0.2 0.4 0.6 0.8 1]  Ns=96  Np=2  BattCapInit=131.82  Tc=1/1000  Vinit=4.221
  SOCto% : Gain  Gain=100
  Scope : Scope
  Stop Simulation : Stop
  lowSOClimit : simulink/Logic and Bit Operations/Compare To Constant  relop=<=  const=5  OutDataTypeStr=boolean
  BatteryVoltage[V] : Outport  VectorParamsAs1DForOutWhenUnconnected=off
  wires:
  Datasheet Battery/1 -> Bus Selector/1
  AmbientTemp[C]/1 -> C2K/1
  Datasheet Battery/2 -> BatteryVoltage[V]/1
  C2K/1 -> Datasheet Battery/2
  SOCto%/1 -> lowSOClimit/1, Scope/1
  Bus Selector/1 -> SOCto%/1  "<BattSoc>"
  LoadCurrent[A]/1 -> Datasheet Battery/1
  lowSOClimit/1 -> Stop Simulation/1

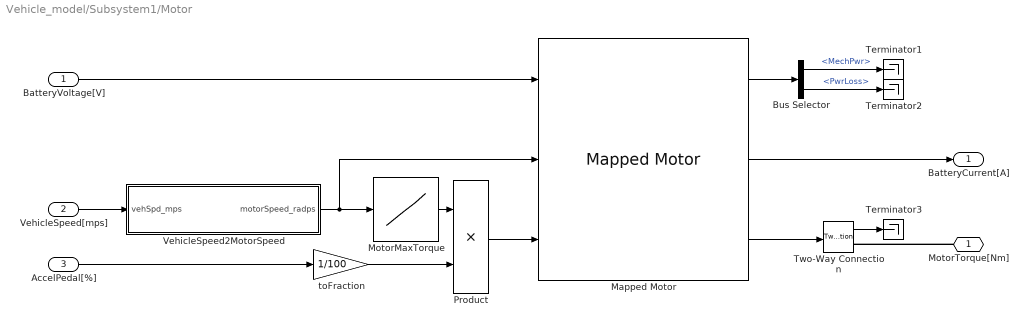
== system Vehicle_model/Subsystem1/Motor ==
  BatteryVoltage[V] : Inport
  VehicleSpeed[mps] : Inport  Port=2
  AccelPedal[%] : Inport  Port=3
  Bus Selector : BusSelector  OutputSignals=MechPwr,PwrLoss
  Mapped Motor : autolibmappedmotor/Mapped Motor  port_config=Speed  param_by=Tabulated torque-speed envelope  w_t=motorSpeedRadPs  T_t=motorMaxTorqueNm  torque_max=.1  power_max=30  Tc=0.02  param_loss=Single efficiency measurement  eff=100  w_eff=375  T_eff=0.08  Piron=0  Pbase=0  w_eff_bp=[-8000 -4000 0 4000 8000]  T_eff_bp=[0 0.03 0.06 0.09]  losses_table=[1.49 1.67 2.21 3.10; 0.42 0.69 1.14 2.03; 0.06 0.24 0.78 1.68; 0.42 0.69 1.14 2.03; 1.49 1.67 2.21 3.10]  efficiency_table=[95 95 95 95; 95 95 95 95; 95 95 95 95; 95 95 95 95; 95 95 95 95]  J=5e-6  b=1e-5  omega_o=0  T_t_extended=[166.666666666667 178.571428571429 192.307692307692 208.333333333333 227.272727272727 250 277.777777777778 312.5 357.142857142857 416.666666666667 500 500 500 500 500 500 500 500 500 500 500 416.666666666667 357.142857142857 312.5 277.777777777778 250 227.272727272727 208.333333333333 192.307692307692 178.571428571429 166.666666666667]  w_t_extended=[-600 -560 -520 -480 -440 -400 -360 -320 -280 -240 -200 -160 -120 -80 -40 0 40 80 120 160 200 240 280 320 360 400 440 480 520 560 600]  KLossIron=0  KLossCopper=0  x_w_eff_vec=[-8000 -4000 0 4000 8000]  x_T_eff_vec=[-0.09 -0.06 -0.03 0 0.03 0.06 0.09]  x_losses_mat=[3.1 2.21 1.67 1.49 1.67 2.21 3.1;2.03 1.14 0.69 0.42 0.69 1.14 2.03;1.68 0.78 0.24 0.06 0.24 0.78 1.68;2.03 1.14 0.69 0.42 0.69 1.14 2.03;3.1 2.21 1.67 1.49 1.67 2.21 3.1]  aMode=aMode
  MotorMaxTorque : Lookup_n-D  NumberOfTableDimensions=1  BreakpointsForDimension1=motorSpeedRadPs  Table=motorMaxTorqueNm  ExtrapMethod=Clip  InternalRulePriority=Speed  RndMeth=Simplest  InputSameDT=on
  Product : Product
  Terminator1 : Terminator
  Terminator2 : Terminator
  Terminator3 : Terminator
  Two-Way Connectio n : TwoWayConnection
  VehicleSpeed2MotorSpeed : Subsystem
  toFraction : Gain  Gain=1/100
  MotorTorque[Nm] : PMIOPort  Side=Right
  BatteryCurrent[A] : Outport  VectorParamsAs1DForOutWhenUnconnected=off
  wires:
  BatteryVoltage[V]/1 -> Mapped Motor/1
  Mapped Motor/2 -> BatteryCurrent[A]/1
  VehicleSpeed[mps]/1 -> VehicleSpeed2MotorSpeed/1(vehSpd_mps)
  VehicleSpeed2MotorSpeed/1(motorSpeed_radps) -> MotorMaxTorque/1, Mapped Motor/2
  Mapped Motor/1 -> Bus Selector/1
  Two-Way Connectio n/1 -> Terminator3/1
  Product/1 -> Mapped Motor/3
  MotorMaxTorque/1 -> Product/1
  AccelPedal[%]/1 -> toFraction/1
  toFraction/1 -> Product/2
  Bus Selector/2 -> Terminator2/1  "<PwrLoss>"
  Bus Selector/1 -> Terminator1/1  "<MechPwr>"
  Mapped Motor/3 -> Two-Way Connectio n/1
  connections:
  MotorTorque[Nm]/RConn1 -- Two-Way Connectio n/RConn1

== system Vehicle_model/Subsystem1/Rear Differential ==
  Axle : autolibsharedcoupling/Torsional Compliance  port_config=Two-way connection  k=axle_k  b=axle_b  theta_o=0  domega_o=0  omega_c=bevAxle_wc  blkID=0  aMode=1
  Open Differential : autolibshareddiff/Open Differential  shaftSwitchMask=To the left of center-line  Ndiff=diffRatio  Jd=.025  bd=1e-3  Jw1=.01  bw1=1e-3  Jw2=.01  bw2=1e-3  omegaw1o=0  omegaw2o=0  maxAbsSpd=5e3  aMode=aMode
  Terminator5 : Terminator
  Terminator6 : Terminator
  Two-Way Connection1 : TwoWayConnection
  Two-Way Connection2 : TwoWayConnection
  AxleTorque[Nm] : PMIOPort  Side=Right
  TorqueInput[Nm] : PMIOPort  Port=2  Side=Left
  wires:
  Open Differential/3 -> Two-Way Connection1/1
  Open Differential/4 -> Terminator5/1
  Open Differential/1 -> Terminator6/1  "Diff"
  Open Differential/2 -> Two-Way Connection2/1
  Two-Way Connection1/1 -> Open Differential/2, Open Differential/3
  Two-Way Connection2/1 -> Open Differential/1
  connections:
  Axle/LConn1 -- Two-Way Connection1/RConn1
  TorqueInput[Nm]/RConn1 -- Two-Way Connection2/RConn1
  AxleTorque[Nm]/RConn1 -- Axle/RConn1

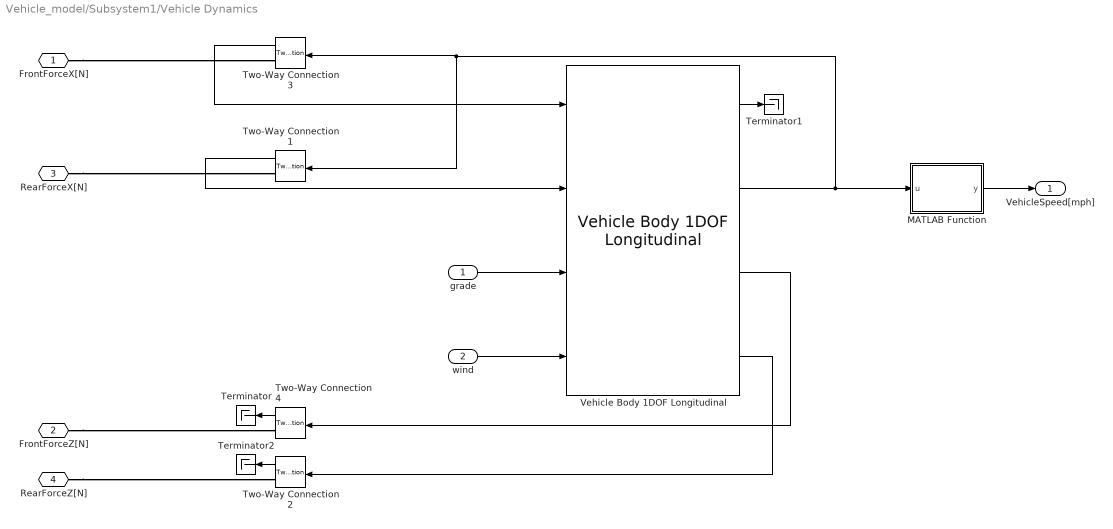
== system Vehicle_model/Subsystem1/Vehicle Dynamics ==
  grade : Inport
  wind : Inport  Port=2
  MATLAB Function : MATLAB Function  TreatAsAtomicUnit=on
  Terminator : Terminator
  Terminator1 : Terminator
  Terminator2 : Terminator
  Two-Way Connection{1..4} (4 alike) : TwoWayConnection
  Vehicle Body 1DOF Longitudinal : autolibshared/Vehicle Body 1DOF Longitudinal  VariantControl=SL  aMode=aMode  NF=2  NR=2  m=1468  a=1.13225  b=1.45575  h=.35  Cd=0.29  Af=2.22  x_o=0  xdot_o=0  Pabs=101325  T=293.15  g=9.81
  FrontForceX[N] : PMIOPort  Side=Left
  FrontForceZ[N] : PMIOPort  Port=2  Side=Left
  RearForceX[N] : PMIOPort  Port=3  Side=Left
  RearForceZ[N] : PMIOPort  Port=4  Side=Left
  VehicleSpeed[mph] : Outport  VectorParamsAs1DForOutWhenUnconnected=off
  wires:
  grade/1 -> Vehicle Body 1DOF Longitudinal/3
  wind/1 -> Vehicle Body 1DOF Longitudinal/4
  Vehicle Body 1DOF Longitudinal/1 -> Terminator1/1
  Vehicle Body 1DOF Longitudinal/3 -> Two-Way Connection4/1
  Vehicle Body 1DOF Longitudinal/4 -> Two-Way Connection2/1
  Two-Way Connection3/1 -> Vehicle Body 1DOF Longitudinal/1
  Two-Way Connection1/1 -> Vehicle Body 1DOF Longitudinal/2
  Two-Way Connection4/1 -> Terminator/1
  Two-Way Connection2/1 -> Terminator2/1
  Vehicle Body 1DOF Longitudinal/2 -> MATLAB Function/1(u), Two-Way Connection1/1, Two-Way Connection3/1
  MATLAB Function/1(y) -> VehicleSpeed[mph]/1
  connections:
  FrontForceX[N]/RConn1 -- Two-Way Connection3/RConn1
  FrontForceZ[N]/RConn1 -- Two-Way Connection4/RConn1
  RearForceX[N]/RConn1 -- Two-Way Connection1/RConn1
  RearForceZ[N]/RConn1 -- Two-Way Connection2/RConn1

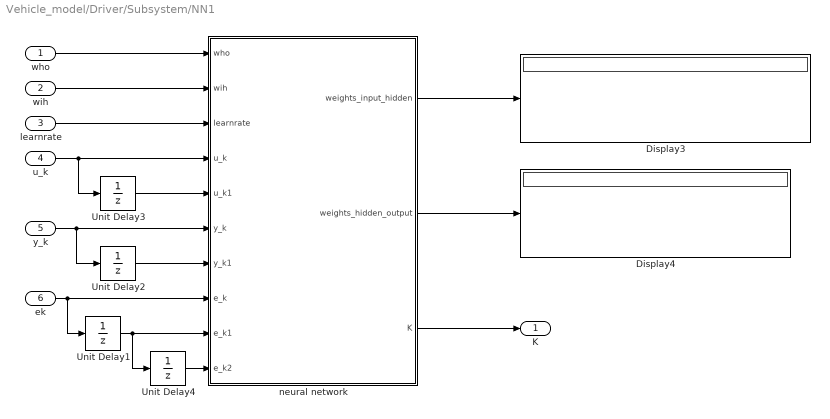
== system Vehicle_model/Driver/Subsystem/NN1 ==
  who : Inport
  wih : Inport  Port=2
  learnrate : Inport  Port=3
  u_k : Inport  Port=4
  y_k : Inport  Port=5
  ek : Inport  Port=6
  Display3 : Display
  Display4 : Display
  Unit Delay{1..4} (4 alike) : UnitDelay  SampleTime=-1  HasFrameUpgradeWarning=on
  neural network : Subsystem
  K : Outport
  wires:
  y_k/1 -> Unit Delay2/1, neural network/6(y_k)
  Unit Delay4/1 -> neural network/10(e_k2)
  Unit Delay3/1 -> neural network/5(u_k1)
  u_k/1 -> Unit Delay3/1, neural network/4(u_k)
  neural network/1(weights_input_hidden) -> Display3/1
  Unit Delay1/1 -> neural network/9(e_k1), Unit Delay4/1
  neural network/2(weights_hidden_output) -> Display4/1
  ek/1 -> neural network/8(e_k), Unit Delay1/1
  Unit Delay2/1 -> neural network/7(y_k1)
  neural network/3(K) -> K/1
  wih/1 -> neural network/2(wih)
  who/1 -> neural network/1(who)
  learnrate/1 -> neural network/3(learnrate)

== system Vehicle_model/Subsystem/Motor/VehicleSpeed2MotorSpeed ==
  vehSpd_mps : Inport
  Gain1 : Gain  Gain=diffRatio
  Gain2 : Gain  Gain=1/wheelRadius
  Signal Specification1 : SignalSpecification  Unit=rad/s
  motorSpeed_radps : Outport  VectorParamsAs1DForOutWhenUnconnected=off
  wires:
  Signal Specification1/1 -> motorSpeed_radps/1
  vehSpd_mps/1 -> Gain1/1
  Gain1/1 -> Gain2/1
  Gain2/1 -> Signal Specification1/1

== system Vehicle_model/Subsystem1/Motor/VehicleSpeed2MotorSpeed ==
  vehSpd_mps : Inport
  Gain1 : Gain  Gain=diffRatio
  Gain2 : Gain  Gain=1/wheelRadius
  Signal Specification1 : SignalSpecification  Unit=rad/s
  motorSpeed_radps : Outport  VectorParamsAs1DForOutWhenUnconnected=off
  wires:
  Signal Specification1/1 -> motorSpeed_radps/1
  vehSpd_mps/1 -> Gain1/1
  Gain1/1 -> Gain2/1
  Gain2/1 -> Signal Specification1/1

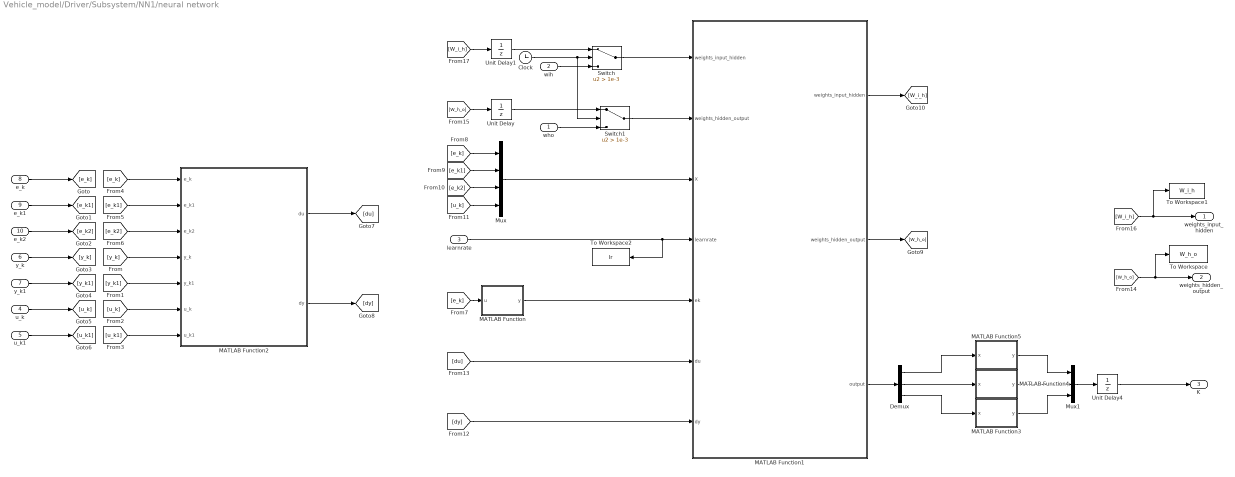
== system Vehicle_model/Driver/Subsystem/NN1/neural network ==
  who : Inport
  wih : Inport  Port=2
  learnrate : Inport  Port=3
  u_k : Inport  Port=4
  u_k1 : Inport  Port=5
  y_k : Inport  Port=6
  y_k1 : Inport  Port=7
  e_k : Inport  Port=8
  e_k1 : Inport  Port=9
  e_k2 : Inport  Port=10
  Clock : Clock
  Demux : Demux  Outputs=3
  MATLAB Function : MATLAB Function  TreatAsAtomicUnit=on
  MATLAB Function1 : MATLAB Function  TreatAsAtomicUnit=on
  MATLAB Function2 : MATLAB Function  TreatAsAtomicUnit=on
  MATLAB Function3 : MATLAB Function  TreatAsAtomicUnit=on
  MATLAB Function4 : MATLAB Function  TreatAsAtomicUnit=on
  MATLAB Function5 : MATLAB Function  TreatAsAtomicUnit=on
  Mux : Mux
  Mux1 : Mux  Inputs=3
  Switch : Switch  Criteria=u2 > Threshold  Threshold=1e-3
  Switch1 : Switch  Criteria=u2 > Threshold  Threshold=1e-3
  To Workspace : ToWorkspace  VariableName=W_h_o  SampleTime=-1
      settings: MaxDataPoints=4  Save2DSignal=2-D array (concatenate along first dimension)
  To Workspace1 : ToWorkspace  VariableName=W_i_h  SampleTime=-1
      settings: MaxDataPoints=4  Save2DSignal=2-D array (concatenate along first dimension)
  To Workspace2 : ToWorkspace  VariableName=lr  SampleTime=-1
      settings: MaxDataPoints=4  Save2DSignal=2-D array (concatenate along first dimension)
  Unit Delay : UnitDelay  SampleTime=-1  HasFrameUpgradeWarning=on
  Unit Delay1 : UnitDelay  SampleTime=-1  HasFrameUpgradeWarning=on
  Unit Delay4 : UnitDelay  SampleTime=-1  HasFrameUpgradeWarning=on
  weights_input_hidden : Outport
  weights_hidden_output : Outport  Port=2
  K : Outport  Port=3
  wires:
  Switch1/1 -> MATLAB Function1/2("weights_hidden_output ")
  Mux/1 -> MATLAB Function1/3(X)
  Unit Delay/1 -> Switch1/1
  wih/1 -> Switch/3
  [e_k1] -> MATLAB Function2/2(e_k1)
  [e_k2] -> MATLAB Function2/3(e_k2)
  learnrate/1 -> MATLAB Function1/4(learnrate), To Workspace2/1
  Switch/1 -> MATLAB Function1/1("weights_input_hidden ")
  who/1 -> Switch1/3
  [y_k] -> MATLAB Function2/4(y_k)
  Clock/1 -> Switch/2, Switch1/2
  Unit Delay1/1 -> Switch/1
  [y_k1] -> MATLAB Function2/5(y_k1)
  [u_k1] -> MATLAB Function2/7(u_k1)
  Demux/1 -> MATLAB Function5/1(x)
  Demux/2 -> MATLAB Function4/1(x)
  Demux/3 -> MATLAB Function3/1(x)
  [W_h_o] -> To Workspace/1, weights_hidden_output/1
  [dy] -> MATLAB Function1/7(dy)
  MATLAB Function/1(y) -> MATLAB Function1/5(ek)
  MATLAB Function3/1(y) -> Mux1/3
  MATLAB Function4/1(y) -> Mux1/2
  MATLAB Function5/1(y) -> Mux1/1
  [u_k] -> MATLAB Function2/6(u_k)
  [du] -> MATLAB Function1/6(du)
  [e_k] -> MATLAB Function2/1(e_k)
  MATLAB Function1/3(output) -> Demux/1
  Mux1/1 -> Unit Delay4/1
  Unit Delay4/1 -> K/1
  e_k/1 -> [e_k]
  e_k1/1 -> [e_k1]
  e_k2/1 -> [e_k2]
  y_k/1 -> [y_k]
  y_k1/1 -> [y_k1]
  u_k/1 -> [u_k]
  u_k1/1 -> [u_k1]
  [e_k] -> MATLAB Function/1(u)
  [e_k] -> Mux/1
  [e_k1] -> Mux/2
  [e_k2] -> Mux/3
  [u_k] -> Mux/4
  MATLAB Function2/1(du) -> [du]
  MATLAB Function2/2(dy) -> [dy]
  MATLAB Function1/2(weights_hidden_output) -> [W_h_o]
  [W_h_o] -> Unit Delay/1
  MATLAB Function1/1(weights_input_hidden) -> [W_i_h]
  [W_i_h] -> To Workspace1/1, weights_input_hidden/1
  [W_i_h] -> Unit Delay1/1

== matlab function Vehicle_model/Subsystem/Vehicle Dynamics/MATLAB Function ==
  data: u input; y output
function y = fcn(u)
if u > 10^5;
    u = 10^5;
elseif u < -10^5;
    u=-10^5;
end
y = u;

== matlab function Vehicle_model/Subsystem1/Vehicle Dynamics/MATLAB Function ==
  data: u input; y output
function y = fcn(u)
if u > 10^5;
    u = 10^5;
elseif u < -10^5;
    u=-10^5;
end
y = u;

== matlab function Vehicle_model/Driver/Subsystem/NN1/neural network/MATLAB Function ==
  data: u input; y output
function y = fcn(u)

y = 0.5*u^2;

== matlab function Vehicle_model/Driver/Subsystem/NN1/neural network/MATLAB Function1 ==
  data: weights_input_hidden output; weights_input_hidden input; weights_hidden_output input; X input; learnrate input; ek input; weights_hidden_output output; du input; dy input; output output size=[3,1]
%%%%%%%%%%%%%%%%%%%%%%%%%%%%%%%%%%%%%%%%%%%%%%%%%%%%%%%%%%%%%%%%%%%%%%%%%%%
% Author: Yassine Kebbati
% Date: 20/12/2019
% Control NN-PID-Autonomous_Driving
%%%%%%%%%%%%%%%%%%%%%%%%%%%%%%%%%%%%%%%%%%%%%%%%%%%%%%%%%%%%%%%%%%%%%%%%%%%

function [weights_input_hidden, weights_hidden_output,output]=gradient(weights_input_hidden,weights_hidden_output,X, learnrate, ek, du,dy)


hidden_layer_in = weights_input_hidden'*X;
hidden_layer_out = sig(hidden_layer_in);



output_layer_in = weights_hidden_output'*hidden_layer_out;

output = output_layer_in;


output_error_term = ek * dy *du;


hidden_error_term = (weights_hidden_output * output_error_term) .* (hidden_layer_out.*(1 - hidden_layer_out));



delta_w_h_o = -learnrate * hidden_layer_out * output_error_term.';

delta_w_i_h = -learnrate * X * hidden_error_term.';


weights_input_hidden =  weights_input_hidden + delta_w_i_h;  

weights_hidden_output =  weights_hidden_output + delta_w_h_o;

== matlab function Vehicle_model/Driver/Subsystem/NN1/neural network/MATLAB Function2 ==
  data: e_k input; du output; e_k1 input; e_k2 input; y_k input; y_k1 input; u_k input; u_k1 input; dy output
%%%%%%%%%%%%%%%%%%%%%%%%%%%%%%%%%%%%%%%%%%%%%%%%%%%%%%%%%%%%%%%%%%%%%%%%%%%
% Author: Yassine Kebbati
% Date: 20/12/2019
% Control NN-PID-Autonomous_Driving
%%%%%%%%%%%%%%%%%%%%%%%%%%%%%%%%%%%%%%%%%%%%%%%%%%%%%%%%%%%%%%%%%%%%%%%%%%%

function [du, dy] = error(e_k, e_k1, e_k2, y_k, y_k1, u_k, u_k1)
T = (1e-3);
du = [(e_k - e_k1); T/2*(e_k- e_k1) ;(e_k - 2*e_k1 + e_k2)/T]; 
%du = [(e_k - e_k1); (e_k - e_k1) ;(e_k - 2*e_k1 + e_k2)];

if (u_k - u_k1)==0
   dy = sign(y_k - y_k1); 
else
    dy = sign((y_k - y_k1)/(u_k - u_k1));
end

== matlab function Vehicle_model/Driver/Subsystem/NN1/neural network/MATLAB Function3 ==
  data: x input; y output
function y = relu(x)

if x>0
    y=x;
else
    y=0;
end

== matlab function Vehicle_model/Driver/Subsystem/NN1/neural network/MATLAB Function4 ==
  data: x input; y output
function y = relu(x)

if x>0
    y=x;
else
    y=0;
end

== matlab function Vehicle_model/Driver/Subsystem/NN1/neural network/MATLAB Function5 ==
  data: x input; y output

function y = relu(x)

if x>0
    y=x;
else
    y=0;
end
